simulink model "test_sonarprua1"  (R2020a)
settings: Solver=VariableStepAuto  StartTime=0.0  StopTime=90  RelTol=1e-3
settings Model: Creator=marco  LastModifiedBy=Marco

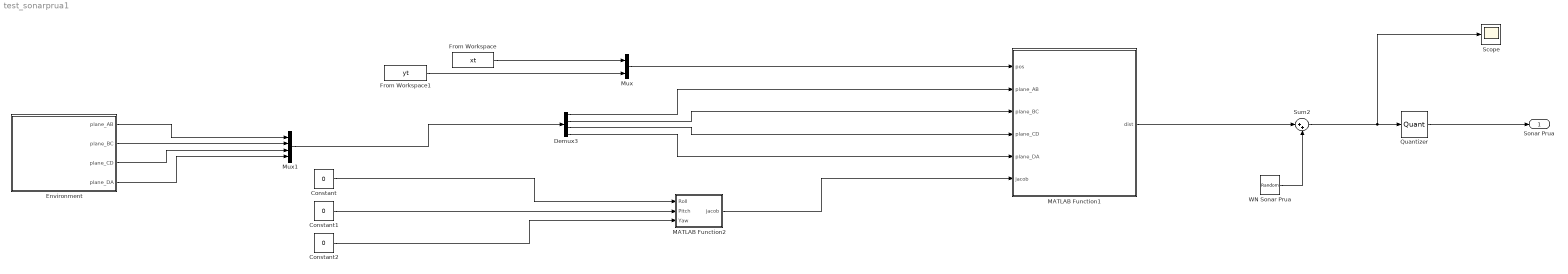
== system test_sonarprua1 ==
  " WN Sonar Prua " : RandomNumber  Variance=0.05  Seed=1234  SampleTime=0.5
  Constant : Constant  Value=0
  Constant1 : Constant  Value=0
  Constant2 : Constant  Value=0
  Demux3 : Demux
  Environment : MATLAB Function  TreatAsAtomicUnit=on
  From Workspace : FromWorkspace  VariableName=xt  SampleTime=0.1
  From Workspace1 : FromWorkspace  VariableName=yt  SampleTime=0.1
  MATLAB Function1 : MATLAB Function  TreatAsAtomicUnit=on  SystemSampleTime=1
  MATLAB Function2 : MATLAB Function  TreatAsAtomicUnit=on
  Mux : Mux  Inputs=2
  Mux1 : Mux
  Quantizer : Quantizer  QuantizationInterval=0.02  LinearizeAsGain=off
  Scope : Scope
  Sum2 : Sum  Inputs=|++
  Sonar Prua : Outport
  wires:
  Demux3/3 -> MATLAB Function1/4(plane_CD)
  Mux/1 -> MATLAB Function1/1(pos)
  Constant2/1 -> MATLAB Function2/3(Yaw)
  Demux3/1 -> MATLAB Function1/2(plane_AB)
  MATLAB Function2/1(jacob) -> MATLAB Function1/6(jacob)
  Demux3/2 -> MATLAB Function1/3(plane_BC)
  Constant/1 -> MATLAB Function2/1(Roll)
  Constant1/1 -> MATLAB Function2/2(Pitch)
  " WN Sonar Prua "/1 -> Sum2/2
  Sum2/1 -> Scope/1, Quantizer/1
  Quantizer/1 -> Sonar Prua/1
  Demux3/4 -> MATLAB Function1/5(plane_DA)
  Mux1/1 -> Demux3/1
  MATLAB Function1/1(dist) -> Sum2/1
  Environment/3(plane_CD) -> Mux1/3
  Environment/4(plane_DA) -> Mux1/4
  Environment/1(plane_AB) -> Mux1/1
  Environment/2(plane_BC) -> Mux1/2
  From Workspace/1 -> Mux/1
  From Workspace1/1 -> Mux/2

== matlab function test_sonarprua1/Environment ==
  data: plane_AB output; plane_BC output; plane_CD output; plane_DA output
function [plane_AB,plane_BC,plane_CD,plane_DA] = fcn()
%% Inizializzazione
% Coordinate degli spigoli del bacino in lat e long fornite dal file
% missionC.m
A= zeros(1,3);
B= zeros(1,3);
C= zeros(1,3);
D= zeros(1,3);
cornerA = [43.781381; 11.282793]; % Lat/Lon [decimal degrees]      
cornerB = [43.780975; 11.283505]; % Lat/Lon [decimal degrees]       
cornerC = [43.780189; 11.282698]; % Lat/Lon [decimal degrees]       
cornerD = [43.780602; 11.281956]; % Lat/Lon [decimal degrees]

% Definizione terna NED con origine (lat0,long0,h0) coincidente al 
% cornerD
coder.extrinsic('evalin', 'wgs84Ellipsoid', 'geodetic2ned');
lat0 = cornerC(1);
lon0 = cornerC(2);
h0 = 0;

%% Conversione ECEF to NED
[A(1),A(2),A(3)] = geodetic2ned(cornerA(1),cornerA(2),0,lat0,lon0,h0,wgs84Ellipsoid);
[B(1),B(2),B(3)] = geodetic2ned(cornerB(1),cornerB(2),0,lat0,lon0,h0,wgs84Ellipsoid);
[C(1),C(2),C(3)] = geodetic2ned(cornerC(1),cornerC(2),0,lat0,lon0,h0,wgs84Ellipsoid);
[D(1),D(2),D(3)] = geodetic2ned(cornerD(1),cornerD(2),0,lat0,lon0,h0,wgs84Ellipsoid);

%% Calcolo delle distanze dalle pareti
% L'equazione del piano corrisponde a quella della retta perché il piano
% delle pareti è verticale, per cui si risolve un sistema lineare:
% l'equazione del piano deve soddisfare il passaggio da due punti.
% Il parametro a è libero, lo poniamo a=1, il parametro c relativo all'asse
% z sarà sempre pari a zero.

% questo è il sistema da risolvere
b = - (B(1)- A(1)) /( B(2) - A(2) );   %AB
d = - A(1) - A(2)*b;

e = - (C(1)-B(1))/(C(2)-B(2));         %BC
f = - B(1) - B(2)*e;

g = - (D(1) - C(1)) / (D(2) - C(2));   %CD
h = - C(1) - C(2)*g;

i = - (A(1) - D(1))/(A(2) - D(2));     %DA
l = -D(1) - D(2)*i;

% syms b d;
% [b d] = solve(A(1)+b*A(2)+d,B(1)+b*B(2)+d,b,d);
a_AB = 1;
b_AB = double(b);
c_AB = 0;
d_AB = double(d);
% 
% syms b d ;
% [b d] = solve(B(1)+b*B(2)+d,C(1)+b*C(2)+d,b,d);
a_BC = 1;
b_BC = double(e);
c_BC = 0;
d_BC = double(f);

a_CD = 1;
b_CD = double(g);
c_CD = 0;
d_CD = double(h);

a_DA = 1;
b_DA = double(i);
c_DA = 0;
d_DA = double(l);


% calcolo dei coefficienti del piano direttamente con la formula esplicita
plane_AB = [a_AB b_AB c_AB d_AB];
plane_BC = [a_BC b_BC c_BC d_BC];
plane_CD = [a_CD b_CD c_CD d_CD];
plane_DA = [a_DA b_DA c_DA d_DA];

== matlab function test_sonarprua1/MATLAB Function1 ==
  data: pos input; plane_AB input; plane_BC input; plane_CD input; plane_DA input; dist output; jacob input
function dist = inter(pos,plane_AB,plane_BC,plane_CD,plane_DA,jacob)
    
    versore_son_body = [1 0 0]';
    versore_son_NED = jacob*versore_son_body;         %versore terna NED sonar sx

    %imposto il sistema per trovare l'intersezione tra la retta con direzione
    %nota e uno dei piani delle pareti del bacino

    t_AB = -(pos(1)+plane_AB(2)*pos(2)+plane_AB(4))/(plane_AB(2)*versore_son_NED(2)+versore_son_NED(1));
    t_BC = -(pos(1)+plane_BC(2)*pos(2)+plane_BC(4))/(plane_BC(2)*versore_son_NED(2)+versore_son_NED(1));
    t_CD = -(pos(1)+plane_CD(2)*pos(2)+plane_CD(4))/(plane_CD(2)*versore_son_NED(2)+versore_son_NED(1));
    t_DA = -(pos(1)+plane_DA(2)*pos(2)+plane_DA(4))/(plane_DA(2)*versore_son_NED(2)+versore_son_NED(1));
    
    
    if t_AB < 0
        t_AB = inf;
    end
    if t_BC < 0
        t_BC = inf;
    end
    if t_CD < 0
        t_CD = inf;
    end
    if t_DA < 0
        t_DA = inf;
    end
           
    dist = min([t_AB t_BC t_CD t_DA]);
end

== matlab function test_sonarprua1/MATLAB Function2 ==
  data: Roll input; jacob output; Pitch input; Yaw input
function jacob  = fcn(Roll,Pitch,Yaw)
 R_x = [1        0              0;
      0 cos(Roll)  sin(Roll);
      0 -sin(Roll) cos(Roll)];
  
R_y = [cos(Pitch) 0 -sin(Pitch);
          0           1         0;
       sin(Pitch) 0 cos(Pitch)];
   
R_z = [cos(Yaw) sin(Yaw) 0;
      -sin(Yaw) cos(Yaw) 0;
          0                 0        1];
      
jaco = (R_z'*R_y');
jacob = jaco*R_x';
end
